simulink model "shapeTracingSawyer"  (R2021a)
settings: Solver=FixedStepAuto  StartTime=0.0  StopTime=12  FixedStep=.01  RelTol=1e-3
values from neighbouring files (symbols this model uses):
  jointPathSegmentMatrix = zeros(length(pathSegments),numJoints,numSamples)    [movimento_sawyer.m]
undefined symbols (not defined in the file or in its folder): B, Spline
libraries: robotcorelib x2, robotmaniplib x1
settings Model: Creator=The MathWorks, Inc.  LastModifiedBy=The MathWorks, Inc.
settings SolverCC: AlgebraicLoopSolver=TrustRegion
settings DataIOCC: ReturnWorkspaceOutputs=off
settings DebuggingCC: SFMachineParentedDataDiag=warning  ArithmeticOperatorsInVariantConditions=warning
settings SFSimCC: CustomCodeUndefinedFunction=UseInterfaceOnly

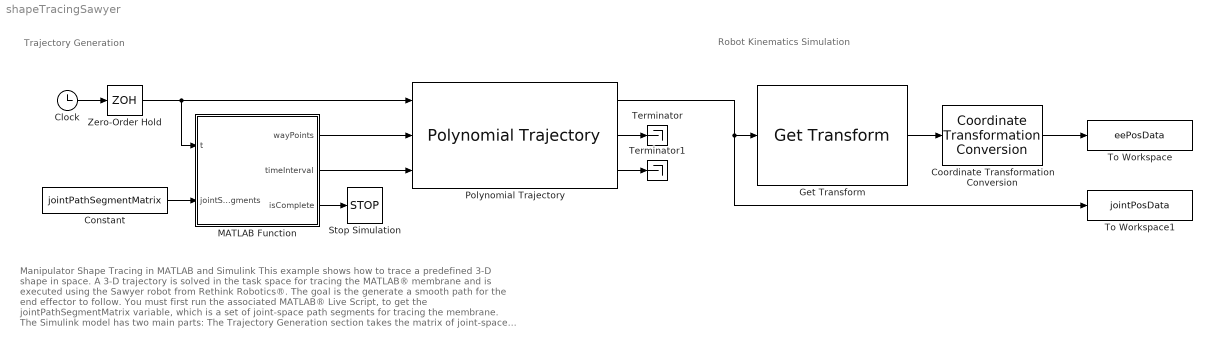
== system shapeTracingSawyer ==
  note: Manipulator Shape Tracing in MATLAB and Simulink
      | This example shows how to trace a predefined 3-D shape in space. A 3-D trajectory is solved in the task space for tracing the MATLAB® membrane and is executed using the Sawyer robot from Rethink Robotics®. The goal is the generate a smooth path for the end effector to follow.
      |
      | You must first run the associated MATLAB® Live Script, to get the jointPathSegmentMatrix variable, which is a set of joint-space path segments for tracing the membrane.
      |
      | The Simulink model has two main parts:
      | The Trajectory Generation section takes the matrix of joint-space path segments, jointPathSegmentMatrix , and converts the segments to a set of discretized joint-space waypoints (joint configurations) at each time step in the simulation using a MATLAB function block. The Polynomial Trajectory Block converts the set of joint configurations to a smoothed B-spline trajectory in time.
      | The Kinematic Simulation section accepts the joint-space waypoints and computes the resulting end-effector position for the robot.
      | Copyright 2018 The MathWorks, Inc.
  note: Trajectory Generation
  note: Robot Kinematics Simulation
  Clock : Clock
  Constant : Constant  Value=jointPathSegmentMatrix
  Coordinate Transformation Conversion : robotcorelib/Coordinate Transformation Conversion  InputRepresentation=Homogeneous Transformation  InputEulerSequence=ZYX  ShowTrVecInputPort=on  OutputRepresentation=Translation Vector  OutputEulerSequence=ZYX  ShowTrVecOutputPort=on  SimulateUsing=Interpreted execution
      settings: SourceProductBaseCode=NV,RO,RR,UV
  Get Transform : robotmaniplib/Get Transform  RigidBodyTree=sawyer  SourceBody=right_hand  TargetBody=base  SimulateUsing=Interpreted execution
  MATLAB Function : MATLAB Function  TreatAsAtomicUnit=on
  Polynomial Trajectory : robotcorelib/Polynomial Trajectory  WaypointSource=External  Waypoints=[ 0, 2, 1, 5, 0; -1, 3, 1, 4, 4 ]  TimePoints=[ 0, 1, 2, 3, 4 ]  TimeInterval=[ 1, 4 ]  Method=B-Spline  ParameterSource=Internal  VelocityBoundaryCondition=zeros( 2, 5 )  AccelerationBoundaryCondition=zeros( 2, 5 )  SimulateUsing=Interpreted execution
  Stop Simulation : Stop
  Terminator : Terminator
  Terminator1 : Terminator
  To Workspace : ToWorkspace  VariableName=eePosData  SaveFormat=Timeseries  SampleTime=-1
  To Workspace1 : ToWorkspace  VariableName=jointPosData  SaveFormat=Timeseries  SampleTime=-1
  Zero-Order Hold : ZeroOrderHold  SampleTime=-1
  wires:
  Polynomial Trajectory/1 -> To Workspace1/1, Get Transform/1
  Clock/1 -> Zero-Order Hold/1
  Get Transform/1 -> Coordinate Transformation Conversion/1
  Coordinate Transformation Conversion/1 -> To Workspace/1
  Polynomial Trajectory/3 -> Terminator1/1
  Polynomial Trajectory/2 -> Terminator/1
  MATLAB Function/1(wayPoints) -> Polynomial Trajectory/2
  MATLAB Function/2(timeInterval) -> Polynomial Trajectory/3
  Constant/1 -> MATLAB Function/2(jointSegments)
  MATLAB Function/3(isComplete) -> Stop Simulation/1
  Zero-Order Hold/1 -> MATLAB Function/1(t), Polynomial Trajectory/1

== matlab function shapeTracingSawyer/MATLAB Function ==
  data: t input; wayPoints output size=[8, numSamples]; jointSegments input; timeInterval output; isComplete output
function [wayPoints, timeInterval, isComplete] = fcn(t, jointSegments)

segmentDuration = 2;
numJoints = 8;
numSegs = size(jointSegments, 1);
numSamples = size(jointSegments, 3);

% Initialize output
wayPoints = zeros(numJoints, numSamples);

% Get current index (indexes from zero)
segIndex = floor(t/segmentDuration);

if (segIndex+1) <= numSegs

    % Define the time interval
    currentStartTime = segIndex*segmentDuration;
    currentEndTime = segIndex*segmentDuration + segmentDuration;
    timeInterval = [currentStartTime currentEndTime];

    % Number of points in the segment
    wayPoints(:,:) = reshape(jointSegments(segIndex + 1, :, :), numJoints, numSamples);
    isComplete = 0;
else
    wayPoints(:,:) = reshape(jointSegments(numSegs, :, :), numJoints, numSamples);
    timeInterval = [0 1];
    isComplete = 1;

end
